simulink subsystem "MotorFOCSL"  (R2024b)
settings: Solver=VariableStepAuto  StartTime=0.0  StopTime=10.0  RelTol=1e-3
values from neighbouring files (symbols this model uses):
  Ts_motor = T_pwm    (= 5e-05)    [s32k344Data.m]
undefined symbols (not defined in the file or in its folder): inverter, pmsm
libraries: autolibpmsminterior x1, mcbplantlib x1, mcbcontrolslib x1
settings Model: Creator=The MathWorks, Inc.  LastModifiedBy=snarayan
settings DebuggingCC: SubsystemReferenceDiagnosticForUnitTest=warning
settings RTWCC: GPUComputeCapability=3.5

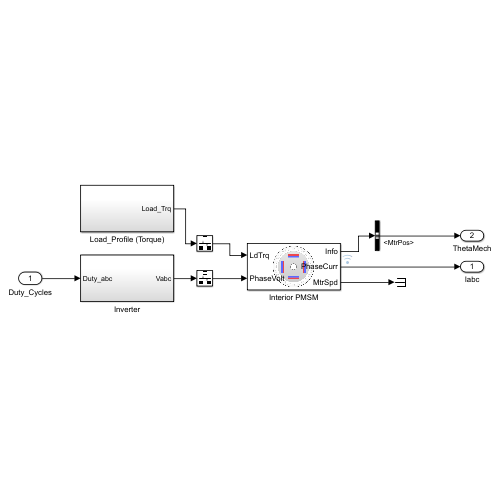
[thumbnail: Simulink's stored preview of the top-level diagram]
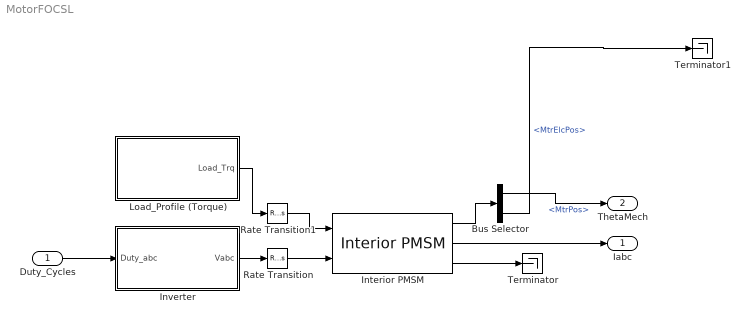
== system MotorFOCSL ==
  Duty_Cycles : Inport
  Bus Selector : BusSelector  OutputSignals=MtrPos,MtrElcPos
  Interior PMSM : autolibpmsminterior/Interior PMSM  port_config=Torque  sim_type=Discrete  Ts=Ts_motor  P=pmsm.p  Rs=pmsm.Rs + inverter.R_board  Ldq=[pmsm.Ld pmsm.Lq]  KConstText=Permanent flux linkage constant (lambda_pm):  lambda_pm=pmsm.FluxPM  Ke=159.9771  mechanical=[pmsm.J, pmsm.B, 0]  idq0=[0 0]  theta_init=0  omega_init=0  KConst=pmsm.FluxPM  lambda_pm_calc=pmsm.FluxPM  Kt=0.07  RefBlkName='autolibpmsminterior/Interior PMSM'  aMode=5
      settings: LibrarySourceBlock=mcblib/Electrical Systems/Motors/Interior PMSM
  Inverter : Subsystem
  Load_Profile (Torque) : Subsystem
  Rate Transition : RateTransition  Deterministic=off  OutPortSampleTime=Ts_motor
  Rate Transition1 : RateTransition  Deterministic=off  OutPortSampleTime=Ts_motor
  Terminator : Terminator
  Terminator1 : Terminator
  Iabc : Outport  VectorParamsAs1DForOutWhenUnconnected=off
  ThetaMech : Outport  Port=2  VectorParamsAs1DForOutWhenUnconnected=off
  wires:
  Inverter/1(Vabc) -> Rate Transition/1
  Duty_Cycles/1 -> Inverter/1(Duty_abc)
  Load_Profile (Torque)/1(Load_Trq) -> Rate Transition1/1
  Rate Transition1/1 -> Interior PMSM/1
  Interior PMSM/3 -> Terminator/1
  Interior PMSM/2 -> Iabc/1
  Rate Transition/1 -> Interior PMSM/2
  Interior PMSM/1 -> Bus Selector/1
  Bus Selector/1 -> ThetaMech/1  "<MtrPos>"
  Bus Selector/2 -> Terminator1/1  "<MtrElcPos>"

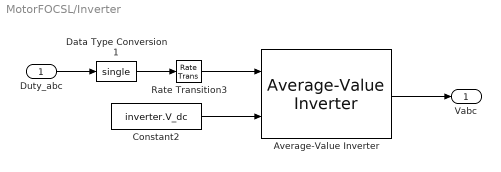
== system MotorFOCSL/Inverter ==
  Duty_abc : Inport
  Average-Value Inverter : mcbplantlib/Average-Value Inverter
  Constant2 : Constant  Value=inverter.V_dc  OutDataTypeStr=single  SampleTime=-1
  Data Type Conversion1 : DataTypeConversion  OutDataTypeStr=single  RndMeth=Simplest  SaturateOnIntegerOverflow=off
  Rate Transition3 : RateTransition  Deterministic=off  OutPortSampleTime=Ts_inverter
  Vabc : Outport  VectorParamsAs1DForOutWhenUnconnected=off
  wires:
  Average-Value Inverter/1 -> Vabc/1
  Rate Transition3/1 -> Average-Value Inverter/1
  Duty_abc/1 -> Data Type Conversion1/1
  Data Type Conversion1/1 -> Rate Transition3/1
  Constant2/1 -> Average-Value Inverter/2

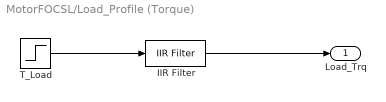
== system MotorFOCSL/Load_Profile (Torque) ==
  IIR Filter : mcbcontrolslib/IIR Filter  VariantControl=Low Pass Filter  VariantSelect=Low-pass  FilterConstantInputType=Specify via dialog  Filter_constant=0.0001  advancedSettings=off  Ts=50e-6  cutOff_freq=0.31834
  T_Load : Step  Time=9  Before=pmsm.T_rated * 0.05  After=pmsm.T_rated * 0.8
  Load_Trq : Outport  VectorParamsAs1DForOutWhenUnconnected=off
  wires:
  IIR Filter/1 -> Load_Trq/1
  T_Load/1 -> IIR Filter/1
